simulink model "TorqueVect"  (R2022a)
settings: Solver=VariableStepAuto  StartTime=0.0  StopTime=32  RelTol=1e-3
PreLoadFcn:
  | run('Parameters\FSE_Parameters.m')
undefined symbols (not defined in the file): BRegenEnabledButton, canChannel, CyalphaLookUp, efficiency, Fz_curve, Fz_scaling_long, gearR, izz, jw, Kd, kd, Ki, ki, Kp, kp, l_f, l_r, lambda, m, Mz_max, N, N_lat, N_long, P_max, pid_kd_lat, pid_kd_long, pid_ki_lat, pid_ki_long, pid_kp_lat, pid_kp_long, R_max, rw, steerR, T_i_max, TC_Decr_Gas, TC_Derivative, TC_Incr_Gas, TC_On, TC_Relay_Off, TC_Relay_On, tireCornerStiffness, Ts, TV_On, TV_Override, velocity_lookup, velocity_lookup_lat, y_ref, yrr_scaling
libraries: simulink x218, slpidlib x135, CarMaker4SL x101, TractionControlLibrary x13, canmsglib x9, canlib x8, TorqueVectoringLibrary x6, simulink_extras x4, PedalConversionLibrary x3, PowerControlLibrary x1
(part 5 of 26)

== system TorqueVect/CarMaker/IPG Vehicle/PowerTrain/PTControl Example/PTControl_ALL_Speedgoat/New TC ==
  lim 1 : Inport
  lim 2 : Inport  Port=2
  lim 3 : Inport  Port=3
  lim 4 : Inport  Port=4
  vx : Inport  Port=5
  w_FL : Inport  Port=6
  w_FR : Inport  Port=7
  w_RL : Inport  Port=8
  w_RR : Inport  Port=9
  Front SR Target : Inport  Port=10
  Rear SR Target : Inport  Port=11
  P_TC : Inport  Port=12
  D_TC : Inport  Port=13
  enable_tc : Inport  Port=14
  rate_h : Inport  Port=15
  rate_l : Inport  Port=16
  Demux1 : Demux
  Gain : Gain  Gain=0.2032/13.39
  Rate Limiter Dynamic{,1..3} (4 alike) : simulink/Discontinuities/Rate Limiter Dynamic
  Reference Generator1 : Subsystem
  Saturation : Saturate  UpperLimit=inf  LowerLimit=0
  Subtract1 : Sum  Inputs=-+
  TC R1 : Subsystem
  TC R2 : Subsystem
  TC R3 : Subsystem
  TC R4 : Subsystem
  Vector Concatenate3 : Concatenate  NumInputs=4
  R1 Demand : Outport
  L1 Demand : Outport  Port=2
  R2 Demand : Outport  Port=3
  L2 Demand : Outport  Port=4
  wires:
  Reference Generator1/1(R1) -> TC R1/1(modified slip ratio reference)
  lim 1/1 -> TC R1/2(lim 1)
  Gain/1 -> Subtract1/2
  Vector Concatenate3/1 -> Gain/1  "omega"
  Subtract1/1 -> Demux1/1
  vx/1 -> Saturation/1
  TC R2/1(Control Effort 1) -> Rate Limiter Dynamic1/2  "MMotorL1Demand"
  w_RL/1 -> Vector Concatenate3/4
  w_RR/1 -> Vector Concatenate3/3
  w_FL/1 -> Vector Concatenate3/2
  w_FR/1 -> Vector Concatenate3/1
  Front SR Target/1 -> Reference Generator1/2(Front SR Target)
  Rear SR Target/1 -> Reference Generator1/3(Rear SR Target)
  lim 2/1 -> TC R2/2(lim 1)
  lim 3/1 -> TC R3/2(lim 1)
  lim 4/1 -> TC R4/2(lim 1)
  Reference Generator1/2(L1) -> TC R2/1(modified slip ratio reference)
  Reference Generator1/3(R2) -> TC R3/1(modified slip ratio reference)
  Reference Generator1/4(L2) -> TC R4/1(modified slip ratio reference)
  P_TC/1 -> TC R2/4(P_TC), TC R4/4(P_TC), TC R3/4(P_TC), TC R1/4(P_TC)
  D_TC/1 -> TC R2/5(D_TC), TC R4/5(D_TC), TC R3/5(D_TC), TC R1/5(D_TC)
  Demux1/1 -> TC R1/3(modified slip ratio measurement)
  Demux1/2 -> TC R2/3(modified slip ratio measurement)
  Demux1/3 -> TC R3/3(modified slip ratio measurement)
  Demux1/4 -> TC R4/3(modified slip ratio measurement)
  TC R1/1(Control Effort 1) -> Rate Limiter Dynamic/2  "MMotorR1Demand"
  Saturation/1 -> Subtract1/1, Reference Generator1/1(x2)
  TC R3/1(Control Effort 1) -> Rate Limiter Dynamic2/2
  TC R4/1(Control Effort 1) -> Rate Limiter Dynamic3/2
  enable_tc/1 -> TC R4/6(enable_tc), TC R2/6(enable_tc), TC R3/6(enable_tc), TC R1/6(enable_tc)
  Rate Limiter Dynamic/1 -> R1 Demand/1
  rate_h/1 -> Rate Limiter Dynamic3/1, Rate Limiter Dynamic2/1, Rate Limiter Dynamic1/1, Rate Limiter Dynamic/1
  rate_l/1 -> Rate Limiter Dynamic/3, Rate Limiter Dynamic3/3, Rate Limiter Dynamic2/3, Rate Limiter Dynamic1/3
  Rate Limiter Dynamic1/1 -> L1 Demand/1
  Rate Limiter Dynamic2/1 -> R2 Demand/1
  Rate Limiter Dynamic3/1 -> L2 Demand/1

== system TorqueVect/CarMaker/IPG Vehicle/PowerTrain/PTControl Example/PTControl_ALL_Speedgoat/PTC ==
  Constant2 : Constant
  Ground : Ground
  Mode_EngineDrive : Constant  Value=4
  Mux : Mux
  OperState_Driving : Constant  Value=4
  PTC MiscOut : Outport  VectorParamsAs1DForOutWhenUnconnected=off
  wires:
  Constant2/1 -> Mux/4  "Ignition"
  Mode_EngineDrive/1 -> Mux/3
  Ground/1 -> Mux/2  "OperationError"
  OperState_Driving/1 -> Mux/1
  Mux/1 -> PTC MiscOut/1

== system TorqueVect/CarMaker/IPG Vehicle/PowerTrain/PTControl Example/PTControl_ALL_Speedgoat/Subsystem ==
  VhclCtrl.PT : Inport
  PTControl_In : Inport  Port=2
  Bus Selector : BusSelector  OutputSignals=VhclCtrl Gas,VhclCtrl Brake
  Bus Selector1 : BusSelector  OutputSignals=Vel_B x,Vel_B y,Omega_B z,Acc_B x,Acc_B y
  Bus Selector2 : BusSelector  OutputSignals=PT:Motor.PT:Motor:Trq,PT:Motor.PT:Motor1:Trq,PT:Motor.PT:Motor2:Trq,PT:Motor.PT:Motor3:Trq,PT:Motor.PT:Motor:rotv,PT:Motor.PT:Motor1:rotv,PT:Motor.PT:Motor2:rotv,PT:Motor.PT:Motor3:rotv,Steer.Driver:Steer:Ang,Steer.Car:SteerAngle:FL,Steer.Car:SteerAngle:FR,PT:PwrSupply:HV1:Pwr
  CAN Configuration : canlib/CAN Configuration  BlockHandle=91645.0002  Device=MathWorks Virtual 1 (Channel 1)  DeviceMenu=MathWorks Virtual 1 (Channel 1)  ObjConstructor=canChannel('MathWorks', 'Virtual 1', 1)  BusSpeed=500000  EnableBitParameters=off  AckMode=Normal
      settings: SourceProductBaseCode=VN
  CAN Pack1 : canmsglib/CAN Pack  MsgList=(none)  MsgName=Wheel Torques  MsgIDType=Standard (11-bit identifier)  MsgIdentifier=600  MsgLength=8  Remote=off  ApplyMinMax=off  BusOutput=off  SignalInfo={ 'FL_Trq', '0', '16', 'LE', 'signed', 'Standard', '0', '1', '0', '-210', '210'; 'FR_Trq', '16', '16', 'LE', 'signed', 'Standard', '0', '1', '0', '-210', '210'; 'RL_Trq', '32', '16', 'LE', 'signed', 'Standard', '0', '1', '0', '-210', '210'; 'RR_Trq', '48', '16', 'LE', 'signed', 'Standard', '0', '1', '0', '-210', '210' }
      settings: SourceProductBaseCode=XP,ME,VN  DataFormat=manually specified signals
  CAN Pack2 : canmsglib/CAN Pack  MsgList=(none)  MsgName=Motor Speeds (rad/s)  MsgIDType=Standard (11-bit identifier)  MsgIdentifier=601  MsgLength=8  Remote=off  ApplyMinMax=off  BusOutput=off  SignalInfo={ 'FL_w', '0', '16', 'LE', 'signed', 'Standard', '0', '1', '0', '-32768', '32767'; 'FR_w', '16', '16', 'LE', 'signed', 'Standard', '0', '1', '0', '-32768', '32767'; 'RL_w', '32', '16', 'LE', 'signed', 'Standard', '0', '1', '0', '-32768', '32767'; 'RR_w', '48', '16', 'LE', 'signed', 'Standard', '0', '1', '0', '-32768', '32767' }
      settings: SourceProductBaseCode=XP,ME,VN  DataFormat=manually specified signals
  CAN Pack3 : canmsglib/CAN Pack  MsgList=(none)  MsgName=CAN Msg  MsgIDType=Standard (11-bit identifier)  MsgIdentifier=602  MsgLength=8  Remote=off  ApplyMinMax=off  BusOutput=off  SignalInfo={ 'Throttle', '0', '8', 'LE', 'unsigned', 'Standard', '0', '1', '0', '0', '100'; 'Brake', '8', '8', 'LE', 'unsigned', 'Standard', '0', '1', '0', '0', '100'; 'Steering Angle', '16', '16', 'LE', 'signed', 'Standard', '0', '1', '0', '-32768', '32767'; 'FL Angle', '32', '16', 'LE', 'signed', 'Standard', '0', '1', '0', '-32768', '32767'; 'FR Angle', '48', '16', 'LE', 'signed', 'Standard', '0', '1', '0', '-32768', '32767' }
      settings: SourceProductBaseCode=XP,ME,VN  DataFormat=manually specified signals
  CAN Pack4 : canmsglib/CAN Pack  MsgList=(none)  MsgName=CAN Msg  MsgIDType=Standard (11-bit identifier)  MsgIdentifier=603  MsgLength=8  Remote=off  ApplyMinMax=off  BusOutput=off  SignalInfo={ 'Vx', '0', '16', 'LE', 'signed', 'Standard', '0', '1', '0', '-32768', '32767'; 'Vy', '16', '16', 'LE', 'signed', 'Standard', '0', '1', '0', '-32768', '32767'; 'nYaw', '32', '16', 'LE', 'signed', 'Standard', '0', '1', '0', '-32768', '32767'; 'Power', '48', '16', 'LE', 'signed', 'Standard', '0', '1', '0', '-8000', '8000' }
      settings: SourceProductBaseCode=XP,ME,VN  DataFormat=manually specified signals
  CAN Pack5 : canmsglib/CAN Pack  Commented=on  MsgList=(none)  MsgName=CAN Msg  MsgIDType=Standard (11-bit identifier)  MsgIdentifier=605  MsgLength=8  Remote=off  ApplyMinMax=off  BusOutput=off  SignalInfo={ 'Pwr', '0', '32', 'LE', 'signed', 'Standard', '0', '1', '0', '-Inf', 'Inf' }
      settings: SourceProductBaseCode=XP,ME,VN  DataFormat=manually specified signals
  CAN Pack6 : canmsglib/CAN Pack  MsgList=(none)  MsgName=CAN Msg  MsgIDType=Standard (11-bit identifier)  MsgIdentifier=604  MsgLength=4  Remote=off  ApplyMinMax=off  BusOutput=off  SignalInfo={ 'Ax', '0', '16', 'LE', 'signed', 'Standard', '0', '1', '0', '-32768', '32767'; 'Ay', '16', '16', 'LE', 'signed', 'Standard', '0', '1', '0', '-32768', '32767' }
      settings: SourceProductBaseCode=XP,ME,VN  DataFormat=manually specified signals
  CAN Transmit1 : canlib/CAN Transmit  BlockHandle=92190.0002  Device=MathWorks Virtual 1 (Channel 1)  DeviceMenu=MathWorks Virtual 1 (Channel 1)  ObjConstructor=canChannel('MathWorks', 'Virtual 1', 1)  EnableEventTransmit=off  EnablePeriodicTransmit=on  MessagePeriod=0.01
      settings: SourceProductBaseCode=VN
  CAN Transmit2 : canlib/CAN Transmit  BlockHandle=92192.0002  Device=MathWorks Virtual 1 (Channel 1)  DeviceMenu=MathWorks Virtual 1 (Channel 1)  ObjConstructor=canChannel('MathWorks', 'Virtual 1', 1)  EnableEventTransmit=off  EnablePeriodicTransmit=on  MessagePeriod=0.01
      settings: SourceProductBaseCode=VN
  CAN Transmit3 : canlib/CAN Transmit  BlockHandle=92194.0002  Device=MathWorks Virtual 1 (Channel 1)  DeviceMenu=MathWorks Virtual 1 (Channel 1)  ObjConstructor=canChannel('MathWorks', 'Virtual 1', 1)  EnableEventTransmit=off  EnablePeriodicTransmit=on  MessagePeriod=0.01
      settings: SourceProductBaseCode=VN
  CAN Transmit4 : canlib/CAN Transmit  Commented=on  BlockHandle=92196.0011  Device=MathWorks Virtual 1 (Channel 1)  DeviceMenu=MathWorks Virtual 1 (Channel 1)  ObjConstructor=canChannel('MathWorks', 'Virtual 1', 1)  EnableEventTransmit=off  EnablePeriodicTransmit=on  MessagePeriod=0.01
      settings: SourceProductBaseCode=VN
  CAN Transmit5 : canlib/CAN Transmit  BlockHandle=92198.0002  Device=MathWorks Virtual 1 (Channel 1)  DeviceMenu=MathWorks Virtual 1 (Channel 1)  ObjConstructor=canChannel('MathWorks', 'Virtual 1', 1)  EnableEventTransmit=off  EnablePeriodicTransmit=on  MessagePeriod=0.01
      settings: SourceProductBaseCode=VN
  CAN Transmit6 : canlib/CAN Transmit  BlockHandle=92200.0002  Device=MathWorks Virtual 1 (Channel 1)  DeviceMenu=MathWorks Virtual 1 (Channel 1)  ObjConstructor=canChannel('MathWorks', 'Virtual 1', 1)  EnableEventTransmit=off  EnablePeriodicTransmit=on  MessagePeriod=0.01
      settings: SourceProductBaseCode=VN
  Gain{,1..3} (4 alike) : Gain  Gain=10
  Gain10 : Gain  Gain=1000
  Gain11 : Gain  Gain=1000
  Gain12 : Gain  Gain=1000
  Gain{8..9,13..15,17..18} (7 alike) : Gain  Gain=100
  Gain16 : Gain  Gain=1/10
  Gain{4..7} (4 alike) : Gain  Gain=30/pi
  Inertial Sensor : CarMaker4SL/Sensors/Inertial Sensor  xname=Param_B00  xstime=Continuous
      settings: SourceProductName=CarMaker4SL
  Rate Transition{,1..18} (19 alike) : RateTransition  OutPortSampleTime=0.001
  Subsystem : Subsystem
  Terminator : Terminator
  <PT:Motor:Trq> : Outport
  <PT:Motor1:Trq> : Outport  Port=2
  <PT:Motor2:Trq> : Outport  Port=3
  <PT:Motor3:Trq> : Outport  Port=4
  wires:
  Inertial Sensor/1 -> Terminator/1
  Inertial Sensor/2 -> Bus Selector1/1
  PTControl_In/1 -> Bus Selector2/1
  VhclCtrl.PT/1 -> Bus Selector/1
  Bus Selector2/1 -> Rate Transition/1  "<PT:Motor:Trq>"
  Bus Selector2/2 -> Rate Transition1/1  "<PT:Motor1:Trq>"
  Bus Selector2/3 -> Rate Transition2/1  "<PT:Motor2:Trq>"
  Bus Selector2/4 -> Rate Transition3/1  "<PT:Motor3:Trq>"
  Bus Selector2/5 -> Rate Transition4/1  "<PT:Motor:rotv>"
  Bus Selector2/6 -> Rate Transition5/1  "<PT:Motor1:rotv>"
  Bus Selector2/7 -> Rate Transition6/1  "<PT:Motor2:rotv>"
  Bus Selector2/8 -> Rate Transition7/1  "<PT:Motor3:rotv>"
  Bus Selector/2 -> Rate Transition9/1  "<VhclCtrl Brake>"
  Bus Selector2/9 -> Rate Transition10/1  "<Driver:Steer:Ang>"
  Bus Selector2/10 -> Rate Transition11/1  "<Car:SteerAngle:FL>"
  Bus Selector2/11 -> Rate Transition12/1  "<Car:SteerAngle:FR>"
  Bus Selector1/1 -> Rate Transition14/1  "<Vel_B x>"
  Bus Selector1/2 -> Rate Transition15/1  "<Vel_B y>"
  Bus Selector1/3 -> Rate Transition16/1  "<Omega_B z>"
  Bus Selector2/12 -> Rate Transition13/1  "<PT:PwrSupply:HV1:Pwr>"
  CAN Pack1/1 -> CAN Transmit1/1
  CAN Pack2/1 -> CAN Transmit2/1
  CAN Pack3/1 -> CAN Transmit3/1
  CAN Pack5/1 -> CAN Transmit4/1
  CAN Pack4/1 -> CAN Transmit5/1
  Subsystem/1(Out1) -> <PT:Motor:Trq>/1
  Subsystem/2(Out2) -> <PT:Motor1:Trq>/1
  Subsystem/3(Out3) -> <PT:Motor2:Trq>/1
  Subsystem/4(Out4) -> <PT:Motor3:Trq>/1
  Rate Transition/1 -> Gain/1
  Rate Transition1/1 -> Gain1/1
  Rate Transition2/1 -> Gain2/1
  Rate Transition3/1 -> Gain3/1
  Rate Transition4/1 -> Gain4/1
  Rate Transition5/1 -> Gain5/1
  Rate Transition6/1 -> Gain6/1
  Rate Transition7/1 -> Gain7/1
  Rate Transition9/1 -> Gain9/1
  Rate Transition10/1 -> Gain10/1
  Rate Transition11/1 -> Gain11/1
  Rate Transition12/1 -> Gain12/1
  Rate Transition13/1 -> Gain16/1
  Rate Transition14/1 -> Gain13/1
  Rate Transition15/1 -> Gain14/1
  Rate Transition16/1 -> Gain15/1
  Bus Selector/1 -> Rate Transition8/1  "<VhclCtrl Gas>"
  Rate Transition8/1 -> Gain8/1
  Gain/1 -> CAN Pack1/1
  Gain1/1 -> CAN Pack1/2
  Gain2/1 -> CAN Pack1/3
  Gain3/1 -> CAN Pack1/4
  Gain6/1 -> CAN Pack2/3
  Gain5/1 -> CAN Pack2/2
  Gain7/1 -> CAN Pack2/4
  Gain4/1 -> CAN Pack2/1
  Gain8/1 -> CAN Pack3/1
  Gain9/1 -> CAN Pack3/2
  Gain10/1 -> CAN Pack3/3
  Gain11/1 -> CAN Pack3/4
  Gain12/1 -> CAN Pack3/5
  Gain13/1 -> CAN Pack4/1
  Gain14/1 -> CAN Pack4/2
  Gain15/1 -> CAN Pack4/3
  Gain16/1 -> CAN Pack4/4, CAN Pack5/1
  Bus Selector1/5 -> Rate Transition18/1  "<Acc_B y>"
  Rate Transition18/1 -> Gain17/1
  Rate Transition17/1 -> Gain18/1
  Gain17/1 -> CAN Pack6/2
  Gain18/1 -> CAN Pack6/1
  Bus Selector1/4 -> Rate Transition17/1  "<Acc_B x>"
  CAN Pack6/1 -> CAN Transmit6/1

== system TorqueVect/CarMaker/IPG Vehicle/PowerTrain/PTControl Example/PTControl_In1/CreateBus PTC Battery ==
  In : Inport
  BusCreator : BusCreator  Inputs=14
  Demux : Demux  Outputs=14
      settings: DisplayOption=none
  Out : Outport  VectorParamsAs1DForOutWhenUnconnected=off
  wires:
  In/1 -> Demux/1
  BusCreator/1 -> Out/1
  Demux/1 -> BusCreator/1  "PTC BattLVIn SOC"
  Demux/2 -> BusCreator/2  "PTC BattLVIn SOH"
  Demux/3 -> BusCreator/3  "PTC BattLVIn Current"
  Demux/4 -> BusCreator/4  "PTC BattLVIn AOC"
  Demux/5 -> BusCreator/5  "PTC BattLVIn Temp"
  Demux/6 -> BusCreator/6  "PTC BattLVIn Energy"
  Demux/7 -> BusCreator/7  "PTC BattLVIn Pwr_max"
  Demux/8 -> BusCreator/8  "PTC BattHVIn SOC"
  Demux/9 -> BusCreator/9  "PTC BattHVIn SOH"
  Demux/10 -> BusCreator/10  "PTC BattHVIn Current"
  Demux/11 -> BusCreator/11  "PTC BattHVIn AOC"
  Demux/12 -> BusCreator/12  "PTC BattHVIn Temp"
  Demux/13 -> BusCreator/13  "PTC BattHVIn Energy"
  Demux/14 -> BusCreator/14  "PTC BattHVIn Pwr_max"

== system TorqueVect/CarMaker/IPG Vehicle/PowerTrain/PTControl Example/PTControl_In1/CreateBus PTC ClutchIn ==
  In : Inport
  BusCreator : BusCreator  Inputs=6
  Demux : Demux  Outputs=6
      settings: DisplayOption=none
  Out : Outport  VectorParamsAs1DForOutWhenUnconnected=off
  wires:
  In/1 -> Demux/1
  BusCreator/1 -> Out/1
  Demux/1 -> BusCreator/1  "PTC ClutchIn Pos"
  Demux/2 -> BusCreator/2  "PTC ClutchIn rotv_in"
  Demux/3 -> BusCreator/3  "PTC ClutchIn rotv_out"
  Demux/4 -> BusCreator/4  "PTC ClutchIn Trq_in"
  Demux/5 -> BusCreator/5  "PTC ClutchIn Trq_out"
  Demux/6 -> BusCreator/6  "PTC ClutchIn i_TrqIn2Out"

== system TorqueVect/CarMaker/IPG Vehicle/PowerTrain/PTControl Example/PTControl_In1/CreateBus PTC Control Units ==
  In : Inport
  BusCreator : BusCreator  Inputs=4
  Demux : Demux
      settings: DisplayOption=none
  Out : Outport  VectorParamsAs1DForOutWhenUnconnected=off
  wires:
  In/1 -> Demux/1
  BusCreator/1 -> Out/1
  Demux/1 -> BusCreator/1  "PTC ECU_Status"
  Demux/2 -> BusCreator/2  "PTC MCU_Status"
  Demux/3 -> BusCreator/3  "PTC TCU_Status"
  Demux/4 -> BusCreator/4  "PTC BCU_Status"

== system TorqueVect/CarMaker/IPG Vehicle/PowerTrain/PTControl Example/PTControl_In1/CreateBus PTC DriveSrcIn ==
  In : Inport
  BusCreator : BusCreator  Inputs=4
  Demux : Demux
      settings: DisplayOption=none
  Out : Outport  VectorParamsAs1DForOutWhenUnconnected=off
  wires:
  In/1 -> Demux/1
  BusCreator/1 -> Out/1
  Demux/1 -> BusCreator/1  "PTC DriveSrcIn_d0 Trq_DriveSrc_trg"
  Demux/2 -> BusCreator/2  "PTC DriveSrcIn_d1 Trq_DriveSrc_trg"
  Demux/3 -> BusCreator/3  "PTC DriveSrcIn_d2 Trq_DriveSrc_trg"
  Demux/4 -> BusCreator/4  "PTC DriveSrcIn_d3 Trq_DriveSrc_trg"

== system TorqueVect/CarMaker/IPG Vehicle/PowerTrain/PTControl Example/PTControl_In1/CreateBus PTC EngineIn ==
  In : Inport
  BusCreator : BusCreator  Inputs=7
  Demux : Demux  Outputs=7
      settings: DisplayOption=none
  Out : Outport  VectorParamsAs1DForOutWhenUnconnected=off
  wires:
  In/1 -> Demux/1
  BusCreator/1 -> Out/1
  Demux/1 -> BusCreator/1  "PTC EngineIn Engine_on"
  Demux/2 -> BusCreator/2  "PTC EngineIn rotv"
  Demux/3 -> BusCreator/3  "PTC EngineIn Trq"
  Demux/4 -> BusCreator/4  "PTC EngineIn TrqDrag"
  Demux/5 -> BusCreator/5  "PTC EngineIn TrqFull"
  Demux/6 -> BusCreator/6  "PTC EngineIn TrqOpt"
  Demux/7 -> BusCreator/7  "PTC EngineIn FuelFlow"

== system TorqueVect/CarMaker/IPG Vehicle/PowerTrain/PTControl Example/PTControl_In1/CreateBus PTC GearBoxIn ==
  In : Inport
  BusCreator : BusCreator  Inputs=20
  Demux : Demux  Outputs=20
      settings: DisplayOption=none
  Out : Outport  VectorParamsAs1DForOutWhenUnconnected=off
  wires:
  In/1 -> Demux/1
  BusCreator/1 -> Out/1
  Demux/1 -> BusCreator/1  "PTC GearBoxIn GearNo"
  Demux/2 -> BusCreator/2  "PTC GearBoxIn GearNo_dis"
  Demux/3 -> BusCreator/3  "PTC GearBoxIn Trq_DriveSrc_trg"
  Demux/4 -> BusCreator/4  "PTC GearBoxIn i"
  Demux/5 -> BusCreator/5  "PTC GearBoxIn rotv_in"
  Demux/6 -> BusCreator/6  "PTC GearBoxIn rotv_out"
  Demux/7 -> BusCreator/7  "PTC GearBoxIn Trq_in"
  Demux/8 -> BusCreator/8  "PTC GearBoxIn Trq_out"
  Demux/9 -> BusCreator/9  "PTC GearBoxIn Clutch Pos"
  Demux/10 -> BusCreator/10  "PTC GearBoxIn Clutch rotv_in"
  Demux/11 -> BusCreator/11  "PTC GearBoxIn Clutch rotv_out"
  Demux/12 -> BusCreator/12  "PTC GearBoxIn Clutch Trq_in"
  Demux/13 -> BusCreator/13  "PTC GearBoxIn Clutch Trq_out"
  Demux/14 -> BusCreator/14  "PTC GearBoxIn Clutch i_TrqIn2Out"
  Demux/15 -> BusCreator/15  "PTC GearBoxIn Clutch_dis Pos"
  Demux/16 -> BusCreator/16  "PTC GearBoxIn Clutch_dis rotv_in"
  Demux/17 -> BusCreator/17  "PTC GearBoxIn Clutch_dis rotv_out"
  Demux/18 -> BusCreator/18  "PTC GearBoxIn Clutch_dis Trq_in"
  Demux/19 -> BusCreator/19  "PTC GearBoxIn Clutch_dis Trq_out"
  Demux/20 -> BusCreator/20  "PTC GearBoxIn Clutch_dis i_TrqIn2Out"

== system TorqueVect/CarMaker/IPG Vehicle/PowerTrain/PTControl Example/PTControl_In1/CreateBus PTC GearBoxM_In0 ==
  In : Inport
  BusCreator : BusCreator  Inputs=20
  Demux : Demux  Outputs=20
      settings: DisplayOption=none
  Out : Outport  VectorParamsAs1DForOutWhenUnconnected=off
  wires:
  In/1 -> Demux/1
  BusCreator/1 -> Out/1
  Demux/1 -> BusCreator/1  "PTC GearBoxM_In0 GearNo"
  Demux/2 -> BusCreator/2  "PTC GearBoxM_In0 GearNo_dis"
  Demux/3 -> BusCreator/3  "PTC GearBoxM_In0 Trq_DriveSrc_trg"
  Demux/4 -> BusCreator/4  "PTC GearBoxM_In0 i"
  Demux/5 -> BusCreator/5  "PTC GearBoxM_In0 rotv_in"
  Demux/6 -> BusCreator/6  "PTC GearBoxM_In0 rotv_out"
  Demux/7 -> BusCreator/7  "PTC GearBoxM_In0 Trq_in"
  Demux/8 -> BusCreator/8  "PTC GearBoxM_In0 Trq_out"
  Demux/9 -> BusCreator/9  "PTC GearBoxM_In0 Clutch Pos"
  Demux/10 -> BusCreator/10  "PTC GearBoxM_In0 Clutch rotv_in"
  Demux/11 -> BusCreator/11  "PTC GearBoxM_In0 Clutch rotv_out"
  Demux/12 -> BusCreator/12  "PTC GearBoxM_In0 Clutch Trq_in"
  Demux/13 -> BusCreator/13  "PTC GearBoxM_In0 Clutch Trq_out"
  Demux/14 -> BusCreator/14  "PTC GearBoxM_In0 Clutch i_TrqIn2Out"
  Demux/15 -> BusCreator/15  "PTC GearBoxM_In0 Clutch_dis Pos"
  Demux/16 -> BusCreator/16  "PTC GearBoxM_In0 Clutch_dis rotv_in"
  Demux/17 -> BusCreator/17  "PTC GearBoxM_In0 Clutch_dis rotv_out"
  Demux/18 -> BusCreator/18  "PTC GearBoxM_In0 Clutch_dis Trq_in"
  Demux/19 -> BusCreator/19  "PTC GearBoxM_In0 Clutch_dis Trq_out"
  Demux/20 -> BusCreator/20  "PTC GearBoxM_In0 Clutch_dis i_TrqIn2Out"

== system TorqueVect/CarMaker/IPG Vehicle/PowerTrain/PTControl Example/PTControl_In1/CreateBus PTC GearBoxM_In1 ==
  In : Inport
  BusCreator : BusCreator  Inputs=20
  Demux : Demux  Outputs=20
      settings: DisplayOption=none
  Out : Outport  VectorParamsAs1DForOutWhenUnconnected=off
  wires:
  In/1 -> Demux/1
  BusCreator/1 -> Out/1
  Demux/1 -> BusCreator/1  "PTC GearBoxM_In1 GearNo"
  Demux/2 -> BusCreator/2  "PTC GearBoxM_In1 GearNo_dis"
  Demux/3 -> BusCreator/3  "PTC GearBoxM_In1 Trq_DriveSrc_trg"
  Demux/4 -> BusCreator/4  "PTC GearBoxM_In1 i"
  Demux/5 -> BusCreator/5  "PTC GearBoxM_In1 rotv_in"
  Demux/6 -> BusCreator/6  "PTC GearBoxM_In1 rotv_out"
  Demux/7 -> BusCreator/7  "PTC GearBoxM_In1 Trq_in"
  Demux/8 -> BusCreator/8  "PTC GearBoxM_In1 Trq_out"
  Demux/9 -> BusCreator/9  "PTC GearBoxM_In1 Clutch Pos"
  Demux/10 -> BusCreator/10  "PTC GearBoxM_In1 Clutch rotv_in"
  Demux/11 -> BusCreator/11  "PTC GearBoxM_In1 Clutch rotv_out"
  Demux/12 -> BusCreator/12  "PTC GearBoxM_In1 Clutch Trq_in"
  Demux/13 -> BusCreator/13  "PTC GearBoxM_In1 Clutch Trq_out"
  Demux/14 -> BusCreator/14  "PTC GearBoxM_In1 Clutch i_TrqIn2Out"
  Demux/15 -> BusCreator/15  "PTC GearBoxM_In1 Clutch_dis Pos"
  Demux/16 -> BusCreator/16  "PTC GearBoxM_In1 Clutch_dis rotv_in"
  Demux/17 -> BusCreator/17  "PTC GearBoxM_In1 Clutch_dis rotv_out"
  Demux/18 -> BusCreator/18  "PTC GearBoxM_In1 Clutch_dis Trq_in"
  Demux/19 -> BusCreator/19  "PTC GearBoxM_In1 Clutch_dis Trq_out"
  Demux/20 -> BusCreator/20  "PTC GearBoxM_In1 Clutch_dis i_TrqIn2Out"

== system TorqueVect/CarMaker/IPG Vehicle/PowerTrain/PTControl Example/PTControl_In1/CreateBus PTC GearBoxM_In2 ==
  In : Inport
  BusCreator : BusCreator  Inputs=20
  Demux : Demux  Outputs=20
      settings: DisplayOption=none
  Out : Outport  VectorParamsAs1DForOutWhenUnconnected=off
  wires:
  In/1 -> Demux/1
  BusCreator/1 -> Out/1
  Demux/1 -> BusCreator/1  "PTC GearBoxM_In2 GearNo"
  Demux/2 -> BusCreator/2  "PTC GearBoxM_In2 GearNo_dis"
  Demux/3 -> BusCreator/3  "PTC GearBoxM_In2 Trq_DriveSrc_trg"
  Demux/4 -> BusCreator/4  "PTC GearBoxM_In2 i"
  Demux/5 -> BusCreator/5  "PTC GearBoxM_In2 rotv_in"
  Demux/6 -> BusCreator/6  "PTC GearBoxM_In2 rotv_out"
  Demux/7 -> BusCreator/7  "PTC GearBoxM_In2 Trq_in"
  Demux/8 -> BusCreator/8  "PTC GearBoxM_In2 Trq_out"
  Demux/9 -> BusCreator/9  "PTC GearBoxM_In2 Clutch Pos"
  Demux/10 -> BusCreator/10  "PTC GearBoxM_In2 Clutch rotv_in"
  Demux/11 -> BusCreator/11  "PTC GearBoxM_In2 Clutch rotv_out"
  Demux/12 -> BusCreator/12  "PTC GearBoxM_In2 Clutch Trq_in"
  Demux/13 -> BusCreator/13  "PTC GearBoxM_In2 Clutch Trq_out"
  Demux/14 -> BusCreator/14  "PTC GearBoxM_In2 Clutch i_TrqIn2Out"
  Demux/15 -> BusCreator/15  "PTC GearBoxM_In2 Clutch_dis Pos"
  Demux/16 -> BusCreator/16  "PTC GearBoxM_In2 Clutch_dis rotv_in"
  Demux/17 -> BusCreator/17  "PTC GearBoxM_In2 Clutch_dis rotv_out"
  Demux/18 -> BusCreator/18  "PTC GearBoxM_In2 Clutch_dis Trq_in"
  Demux/19 -> BusCreator/19  "PTC GearBoxM_In2 Clutch_dis Trq_out"
  Demux/20 -> BusCreator/20  "PTC GearBoxM_In2 Clutch_dis i_TrqIn2Out"

== system TorqueVect/CarMaker/IPG Vehicle/PowerTrain/PTControl Example/PTControl_In1/CreateBus PTC GearBoxM_In3 ==
  In : Inport
  BusCreator : BusCreator  Inputs=20
  Demux : Demux  Outputs=20
      settings: DisplayOption=none
  Out : Outport  VectorParamsAs1DForOutWhenUnconnected=off
  wires:
  In/1 -> Demux/1
  BusCreator/1 -> Out/1
  Demux/1 -> BusCreator/1  "PTC GearBoxM_In3 GearNo"
  Demux/2 -> BusCreator/2  "PTC GearBoxM_In3 GearNo_dis"
  Demux/3 -> BusCreator/3  "PTC GearBoxM_In3 Trq_DriveSrc_trg"
  Demux/4 -> BusCreator/4  "PTC GearBoxM_In3 i"
  Demux/5 -> BusCreator/5  "PTC GearBoxM_In3 rotv_in"
  Demux/6 -> BusCreator/6  "PTC GearBoxM_In3 rotv_out"
  Demux/7 -> BusCreator/7  "PTC GearBoxM_In3 Trq_in"
  Demux/8 -> BusCreator/8  "PTC GearBoxM_In3 Trq_out"
  Demux/9 -> BusCreator/9  "PTC GearBoxM_In3 Clutch Pos"
  Demux/10 -> BusCreator/10  "PTC GearBoxM_In3 Clutch rotv_in"
  Demux/11 -> BusCreator/11  "PTC GearBoxM_In3 Clutch rotv_out"
  Demux/12 -> BusCreator/12  "PTC GearBoxM_In3 Clutch Trq_in"
  Demux/13 -> BusCreator/13  "PTC GearBoxM_In3 Clutch Trq_out"
  Demux/14 -> BusCreator/14  "PTC GearBoxM_In3 Clutch i_TrqIn2Out"
  Demux/15 -> BusCreator/15  "PTC GearBoxM_In3 Clutch_dis Pos"
  Demux/16 -> BusCreator/16  "PTC GearBoxM_In3 Clutch_dis rotv_in"
  Demux/17 -> BusCreator/17  "PTC GearBoxM_In3 Clutch_dis rotv_out"
  Demux/18 -> BusCreator/18  "PTC GearBoxM_In3 Clutch_dis Trq_in"
  Demux/19 -> BusCreator/19  "PTC GearBoxM_In3 Clutch_dis Trq_out"
  Demux/20 -> BusCreator/20  "PTC GearBoxM_In3 Clutch_dis i_TrqIn2Out"

== system TorqueVect/CarMaker/IPG Vehicle/PowerTrain/PTControl Example/PTControl_In1/CreateBus PTC ISGIn ==
  In : Inport
  BusCreator : BusCreator  Inputs=9
  Demux : Demux  Outputs=9
      settings: DisplayOption=none
  Out : Outport  VectorParamsAs1DForOutWhenUnconnected=off
  wires:
  In/1 -> Demux/1
  BusCreator/1 -> Out/1
  Demux/1 -> BusCreator/1  "PTC ISGIn rotv"
  Demux/2 -> BusCreator/2  "PTC ISGIn Trq"
  Demux/3 -> BusCreator/3  "PTC ISGIn TrqMot_max"
  Demux/4 -> BusCreator/4  "PTC ISGIn TrqGen_max"
  Demux/5 -> BusCreator/5  "PTC ISGIn PwrElec"
  Demux/6 -> BusCreator/6  "PTC ISGIn i_M2W_FL"
  Demux/7 -> BusCreator/7  "PTC ISGIn i_M2W_FR"
  Demux/8 -> BusCreator/8  "PTC ISGIn i_M2W_RL"
  Demux/9 -> BusCreator/9  "PTC ISGIn i_M2W_RR"

== system TorqueVect/CarMaker/IPG Vehicle/PowerTrain/PTControl Example/PTControl_In1/CreateBus PTC MotorIn0 ==
  In : Inport
  BusCreator : BusCreator  Inputs=9
  Demux : Demux  Outputs=9
      settings: DisplayOption=none
  Out : Outport  VectorParamsAs1DForOutWhenUnconnected=off
  wires:
  In/1 -> Demux/1
  BusCreator/1 -> Out/1
  Demux/1 -> BusCreator/1  "PTC MotorIn0 rotv"
  Demux/2 -> BusCreator/2  "PTC MotorIn0 Trq"
  Demux/3 -> BusCreator/3  "PTC MotorIn0 TrqMot_max"
  Demux/4 -> BusCreator/4  "PTC MotorIn0 TrqGen_max"
  Demux/5 -> BusCreator/5  "PTC MotorIn0 PwrElec"
  Demux/6 -> BusCreator/6  "PTC MotorIn0 i_M2W_FL"
  Demux/7 -> BusCreator/7  "PTC MotorIn0 i_M2W_FR"
  Demux/8 -> BusCreator/8  "PTC MotorIn0 i_M2W_RL"
  Demux/9 -> BusCreator/9  "PTC MotorIn0 i_M2W_RR"

== system TorqueVect/CarMaker/IPG Vehicle/PowerTrain/PTControl Example/PTControl_In1/CreateBus PTC MotorIn1 ==
  In : Inport
  BusCreator : BusCreator  Inputs=9
  Demux : Demux  Outputs=9
      settings: DisplayOption=none
  Out : Outport  VectorParamsAs1DForOutWhenUnconnected=off
  wires:
  In/1 -> Demux/1
  BusCreator/1 -> Out/1
  Demux/1 -> BusCreator/1  "PTC MotorIn1 rotv"
  Demux/2 -> BusCreator/2  "PTC MotorIn1 Trq"
  Demux/3 -> BusCreator/3  "PTC MotorIn1 TrqMot_max"
  Demux/4 -> BusCreator/4  "PTC MotorIn1 TrqGen_max"
  Demux/5 -> BusCreator/5  "PTC MotorIn1 PwrElec"
  Demux/6 -> BusCreator/6  "PTC MotorIn1 i_M2W_FL"
  Demux/7 -> BusCreator/7  "PTC MotorIn1 i_M2W_FR"
  Demux/8 -> BusCreator/8  "PTC MotorIn1 i_M2W_RL"
  Demux/9 -> BusCreator/9  "PTC MotorIn1 i_M2W_RR"

== system TorqueVect/CarMaker/IPG Vehicle/PowerTrain/PTControl Example/PTControl_In1/CreateBus PTC MotorIn2 ==
  In : Inport
  BusCreator : BusCreator  Inputs=9
  Demux : Demux  Outputs=9
      settings: DisplayOption=none
  Out : Outport  VectorParamsAs1DForOutWhenUnconnected=off
  wires:
  In/1 -> Demux/1
  BusCreator/1 -> Out/1
  Demux/1 -> BusCreator/1  "PTC MotorIn2 rotv"
  Demux/2 -> BusCreator/2  "PTC MotorIn2 Trq"
  Demux/3 -> BusCreator/3  "PTC MotorIn2 TrqMot_max"
  Demux/4 -> BusCreator/4  "PTC MotorIn2 TrqGen_max"
  Demux/5 -> BusCreator/5  "PTC MotorIn2 PwrElec"
  Demux/6 -> BusCreator/6  "PTC MotorIn2 i_M2W_FL"
  Demux/7 -> BusCreator/7  "PTC MotorIn2 i_M2W_FR"
  Demux/8 -> BusCreator/8  "PTC MotorIn2 i_M2W_RL"
  Demux/9 -> BusCreator/9  "PTC MotorIn2 i_M2W_RR"

== system TorqueVect/CarMaker/IPG Vehicle/PowerTrain/PTControl Example/PTControl_In1/CreateBus PTC MotorIn3 ==
  In : Inport
  BusCreator : BusCreator  Inputs=9
  Demux : Demux  Outputs=9
      settings: DisplayOption=none
  Out : Outport  VectorParamsAs1DForOutWhenUnconnected=off
  wires:
  In/1 -> Demux/1
  BusCreator/1 -> Out/1
  Demux/1 -> BusCreator/1  "PTC MotorIn3 rotv"
  Demux/2 -> BusCreator/2  "PTC MotorIn3 Trq"
  Demux/3 -> BusCreator/3  "PTC MotorIn3 TrqMot_max"
  Demux/4 -> BusCreator/4  "PTC MotorIn3 TrqGen_max"
  Demux/5 -> BusCreator/5  "PTC MotorIn3 PwrElec"
  Demux/6 -> BusCreator/6  "PTC MotorIn3 i_M2W_FL"
  Demux/7 -> BusCreator/7  "PTC MotorIn3 i_M2W_FR"
  Demux/8 -> BusCreator/8  "PTC MotorIn3 i_M2W_RL"
  Demux/9 -> BusCreator/9  "PTC MotorIn3 i_M2W_RR"

== system TorqueVect/CarMaker/IPG Vehicle/PowerTrain/PTControl Example/PTControl_In1/CreateBus PTC PwrSupplyIn ==
  In : Inport
  BusCreator : BusCreator  Inputs=12
  Demux : Demux  Outputs=12
      settings: DisplayOption=none
  Out : Outport  VectorParamsAs1DForOutWhenUnconnected=off
  wires:
  In/1 -> Demux/1
  BusCreator/1 -> Out/1
  Demux/1 -> BusCreator/1  "PTC PwrSupplyIn Pwr_LV"
  Demux/2 -> BusCreator/2  "PTC PwrSupplyIn Pwr_HV1"
  Demux/3 -> BusCreator/3  "PTC PwrSupplyIn Pwr_HV2"
  Demux/4 -> BusCreator/4  "PTC PwrSupplyIn Voltage_LV"
  Demux/5 -> BusCreator/5  "PTC PwrSupplyIn Voltage_HV1"
  Demux/6 -> BusCreator/6  "PTC PwrSupplyIn Voltage_HV2"
  Demux/7 -> BusCreator/7  "PTC PwrSupplyIn Pwr_HV1toLV"
  Demux/8 -> BusCreator/8  "PTC PwrSupplyIn Pwr_HV1toHV2"
  Demux/9 -> BusCreator/9  "PTC PwrSupplyIn Pwr_HV1toLV_max"
  Demux/10 -> BusCreator/10  "PTC PwrSupplyIn Pwr_HV1toHV2_max"
  Demux/11 -> BusCreator/11  "PTC PwrSupplyIn Eta_HV1toLV"
  Demux/12 -> BusCreator/12  "PTC PwrSupplyIn Eta_HV1toHV2"

== system TorqueVect/CarMaker/IPG Vehicle/PowerTrain/PTControl Example/PTControl_In1/CreateBus PTC Vehicle Ctrl ==
  In : Inport
  BusCreator : BusCreator  Inputs=8
  Demux : Demux  Outputs=8
      settings: DisplayOption=none
  Out : Outport  VectorParamsAs1DForOutWhenUnconnected=off
  wires:
  In/1 -> Demux/1
  BusCreator/1 -> Out/1
  Demux/1 -> BusCreator/1  "PTC Key"
  Demux/2 -> BusCreator/2  "PTC SST"
  Demux/3 -> BusCreator/3  "PTC SelectorCtrl"
  Demux/4 -> BusCreator/4  "PTC GearNoTrg"
  Demux/5 -> BusCreator/5  "PTC Clutch"
  Demux/6 -> BusCreator/6  "PTC Gas"
  Demux/7 -> BusCreator/7  "PTC Brake"
  Demux/8 -> BusCreator/8  "PTC Velocity"

== system TorqueVect/CarMaker/IPG Vehicle/PowerTrain/PTControl Example/PTControl_In1/CreateBus PTC WheelIn ==
  In : Inport
  BusCreator : BusCreator  Inputs=4
  Demux : Demux
      settings: DisplayOption=none
  Out : Outport  VectorParamsAs1DForOutWhenUnconnected=off
  wires:
  In/1 -> Demux/1
  BusCreator/1 -> Out/1
  Demux/1 -> BusCreator/1  "PTC WheelIn_FL Trq_BrakeReg_trg"
  Demux/2 -> BusCreator/2  "PTC WheelIn_FR Trq_BrakeReg_trg"
  Demux/3 -> BusCreator/3  "PTC WheelIn_RL Trq_BrakeReg_trg"
  Demux/4 -> BusCreator/4  "PTC WheelIn_RR Trq_BrakeReg_trg"

== system TorqueVect/CarMaker/IPG Vehicle/PowerTrain/PTControl Example/PTControl_In1/CreateBus PTC_Cfg Battery ==
  In : Inport
  BusCreator : BusCreator  Inputs=8
  Demux : Demux  Outputs=8
      settings: DisplayOption=none
  Out : Outport  VectorParamsAs1DForOutWhenUnconnected=off
  wires:
  In/1 -> Demux/1
  BusCreator/1 -> Out/1
  Demux/1 -> BusCreator/1  "PTC_Cfg BattLV SOC_min"
  Demux/2 -> BusCreator/2  "PTC_Cfg BattLV SOC_max"
  Demux/3 -> BusCreator/3  "PTC_Cfg BattLV Capacity"
  Demux/4 -> BusCreator/4  "PTC_Cfg BattLV Voltage"
  Demux/5 -> BusCreator/5  "PTC_Cfg BattHV SOC_min"
  Demux/6 -> BusCreator/6  "PTC_Cfg BattHV SOC_max"
  Demux/7 -> BusCreator/7  "PTC_Cfg BattHV Capacity"
  Demux/8 -> BusCreator/8  "PTC_Cfg BattHV Voltage"

== system TorqueVect/CarMaker/IPG Vehicle/PowerTrain/PTControl Example/PTControl_In1/CreateBus PTC_Cfg Engine ==
  In : Inport
  BusCreator : BusCreator  Inputs=4
  Demux : Demux
      settings: DisplayOption=none
  Out : Outport  VectorParamsAs1DForOutWhenUnconnected=off
  wires:
  In/1 -> Demux/1
  BusCreator/1 -> Out/1
  Demux/1 -> BusCreator/1  "PTC_Cfg Engine Fuel_l2kWh"
  Demux/2 -> BusCreator/2  "PTC_Cfg Engine rotv_max"
  Demux/3 -> BusCreator/3  "PTC_Cfg Engine rotv_idle"
  Demux/4 -> BusCreator/4  "PTC_Cfg Engine rotv_opt"

== system TorqueVect/CarMaker/IPG Vehicle/PowerTrain/PTControl Example/PTControl_In1/CreateBus PTC_Cfg GearBox ==
  In : Inport
  BusCreator : BusCreator  Inputs=38
  Demux : Demux  Outputs=38
      settings: DisplayOption=none
  Out : Outport  VectorParamsAs1DForOutWhenUnconnected=off
  wires:
  In/1 -> Demux/1
  BusCreator/1 -> Out/1
  Demux/1 -> BusCreator/1  "PTC_Cfg GearBox GBKind"
  Demux/2 -> BusCreator/2  "PTC_Cfg GearBox ClKind"
  Demux/3 -> BusCreator/3  "PTC_Cfg GearBox nFGears"
  Demux/4 -> BusCreator/4  "PTC_Cfg GearBox iFGear0"
  Demux/5 -> BusCreator/5  "PTC_Cfg GearBox iFGear1"
  Demux/6 -> BusCreator/6  "PTC_Cfg GearBox iFGear2"
  Demux/7 -> BusCreator/7  "PTC_Cfg GearBox iFGear3"
  Demux/8 -> BusCreator/8  "PTC_Cfg GearBox iFGear4"
  Demux/9 -> BusCreator/9  "PTC_Cfg GearBox iFGear5"
  Demux/10 -> BusCreator/10  "PTC_Cfg GearBox iFGear6"
  Demux/11 -> BusCreator/11  "PTC_Cfg GearBox iFGear7"
  Demux/12 -> BusCreator/12  "PTC_Cfg GearBox iFGear8"
  Demux/13 -> BusCreator/13  "PTC_Cfg GearBox iFGear9"
  Demux/14 -> BusCreator/14  "PTC_Cfg GearBox iFGear10"
  Demux/15 -> BusCreator/15  "PTC_Cfg GearBox iFGear11"
  Demux/16 -> BusCreator/16  "PTC_Cfg GearBox iFGear12"
  Demux/17 -> BusCreator/17  "PTC_Cfg GearBox iFGear13"
  Demux/18 -> BusCreator/18  "PTC_Cfg GearBox iFGear14"
  Demux/19 -> BusCreator/19  "PTC_Cfg GearBox iFGear15"
  Demux/20 -> BusCreator/20  "PTC_Cfg GearBox iFGear16"
  Demux/21 -> BusCreator/21  "PTC_Cfg GearBox nBGears"
  Demux/22 -> BusCreator/22  "PTC_Cfg GearBox iBGear0"
  Demux/23 -> BusCreator/23  "PTC_Cfg GearBox iBGear1"
  Demux/24 -> BusCreator/24  "PTC_Cfg GearBox iBGear2"
  Demux/25 -> BusCreator/25  "PTC_Cfg GearBox iBGear3"
  Demux/26 -> BusCreator/26  "PTC_Cfg GearBox iBGear4"
  Demux/27 -> BusCreator/27  "PTC_Cfg GearBox iBGear5"
  Demux/28 -> BusCreator/28  "PTC_Cfg GearBox iBGear6"
  Demux/29 -> BusCreator/29  "PTC_Cfg GearBox iBGear7"
  Demux/30 -> BusCreator/30  "PTC_Cfg GearBox iBGear8"
  Demux/31 -> BusCreator/31  "PTC_Cfg GearBox iBGear9"
  Demux/32 -> BusCreator/32  "PTC_Cfg GearBox iBGear10"
  Demux/33 -> BusCreator/33  "PTC_Cfg GearBox iBGear11"
  Demux/34 -> BusCreator/34  "PTC_Cfg GearBox iBGear12"
  Demux/35 -> BusCreator/35  "PTC_Cfg GearBox iBGear13"
  Demux/36 -> BusCreator/36  "PTC_Cfg GearBox iBGear14"
  Demux/37 -> BusCreator/37  "PTC_Cfg GearBox iBGear15"
  Demux/38 -> BusCreator/38  "PTC_Cfg GearBox iBGear16"

== system TorqueVect/CarMaker/IPG Vehicle/PowerTrain/PTControl Example/PTControl_In1/CreateBus PTC_Cfg GearBoxM0 ==
  In : Inport
  BusCreator : BusCreator  Inputs=38
  Demux : Demux  Outputs=38
      settings: DisplayOption=none
  Out : Outport  VectorParamsAs1DForOutWhenUnconnected=off
  wires:
  In/1 -> Demux/1
  BusCreator/1 -> Out/1
  Demux/1 -> BusCreator/1  "PTC_Cfg GearBoxM0 GBKind"
  Demux/2 -> BusCreator/2  "PTC_Cfg GearBoxM0 ClKind"
  Demux/3 -> BusCreator/3  "PTC_Cfg GearBoxM0 nFGears"
  Demux/4 -> BusCreator/4  "PTC_Cfg GearBoxM0 iFGear0"
  Demux/5 -> BusCreator/5  "PTC_Cfg GearBoxM0 iFGear1"
  Demux/6 -> BusCreator/6  "PTC_Cfg GearBoxM0 iFGear2"
  Demux/7 -> BusCreator/7  "PTC_Cfg GearBoxM0 iFGear3"
  Demux/8 -> BusCreator/8  "PTC_Cfg GearBoxM0 iFGear4"
  Demux/9 -> BusCreator/9  "PTC_Cfg GearBoxM0 iFGear5"
  Demux/10 -> BusCreator/10  "PTC_Cfg GearBoxM0 iFGear6"
  Demux/11 -> BusCreator/11  "PTC_Cfg GearBoxM0 iFGear7"
  Demux/12 -> BusCreator/12  "PTC_Cfg GearBoxM0 iFGear8"
  Demux/13 -> BusCreator/13  "PTC_Cfg GearBoxM0 iFGear9"
  Demux/14 -> BusCreator/14  "PTC_Cfg GearBoxM0 iFGear10"
  Demux/15 -> BusCreator/15  "PTC_Cfg GearBoxM0 iFGear11"
  Demux/16 -> BusCreator/16  "PTC_Cfg GearBoxM0 iFGear12"
  Demux/17 -> BusCreator/17  "PTC_Cfg GearBoxM0 iFGear13"
  Demux/18 -> BusCreator/18  "PTC_Cfg GearBoxM0 iFGear14"
  Demux/19 -> BusCreator/19  "PTC_Cfg GearBoxM0 iFGear15"
  Demux/20 -> BusCreator/20  "PTC_Cfg GearBoxM0 iFGear16"
  Demux/21 -> BusCreator/21  "PTC_Cfg GearBoxM0 nBGears"
  Demux/22 -> BusCreator/22  "PTC_Cfg GearBoxM0 iBGear0"
  Demux/23 -> BusCreator/23  "PTC_Cfg GearBoxM0 iBGear1"
  Demux/24 -> BusCreator/24  "PTC_Cfg GearBoxM0 iBGear2"
  Demux/25 -> BusCreator/25  "PTC_Cfg GearBoxM0 iBGear3"
  Demux/26 -> BusCreator/26  "PTC_Cfg GearBoxM0 iBGear4"
  Demux/27 -> BusCreator/27  "PTC_Cfg GearBoxM0 iBGear5"
  Demux/28 -> BusCreator/28  "PTC_Cfg GearBoxM0 iBGear6"
  Demux/29 -> BusCreator/29  "PTC_Cfg GearBoxM0 iBGear7"
  Demux/30 -> BusCreator/30  "PTC_Cfg GearBoxM0 iBGear8"
  Demux/31 -> BusCreator/31  "PTC_Cfg GearBoxM0 iBGear9"
  Demux/32 -> BusCreator/32  "PTC_Cfg GearBoxM0 iBGear10"
  Demux/33 -> BusCreator/33  "PTC_Cfg GearBoxM0 iBGear11"
  Demux/34 -> BusCreator/34  "PTC_Cfg GearBoxM0 iBGear12"
  Demux/35 -> BusCreator/35  "PTC_Cfg GearBoxM0 iBGear13"
  Demux/36 -> BusCreator/36  "PTC_Cfg GearBoxM0 iBGear14"
  Demux/37 -> BusCreator/37  "PTC_Cfg GearBoxM0 iBGear15"
  Demux/38 -> BusCreator/38  "PTC_Cfg GearBoxM0 iBGear16"

== system TorqueVect/CarMaker/IPG Vehicle/PowerTrain/PTControl Example/PTControl_In1/CreateBus PTC_Cfg GearBoxM1 ==
  In : Inport
  BusCreator : BusCreator  Inputs=38
  Demux : Demux  Outputs=38
      settings: DisplayOption=none
  Out : Outport  VectorParamsAs1DForOutWhenUnconnected=off
  wires:
  In/1 -> Demux/1
  BusCreator/1 -> Out/1
  Demux/1 -> BusCreator/1  "PTC_Cfg GearBoxM1 GBKind"
  Demux/2 -> BusCreator/2  "PTC_Cfg GearBoxM1 ClKind"
  Demux/3 -> BusCreator/3  "PTC_Cfg GearBoxM1 nFGears"
  Demux/4 -> BusCreator/4  "PTC_Cfg GearBoxM1 iFGear0"
  Demux/5 -> BusCreator/5  "PTC_Cfg GearBoxM1 iFGear1"
  Demux/6 -> BusCreator/6  "PTC_Cfg GearBoxM1 iFGear2"
  Demux/7 -> BusCreator/7  "PTC_Cfg GearBoxM1 iFGear3"
  Demux/8 -> BusCreator/8  "PTC_Cfg GearBoxM1 iFGear4"
  Demux/9 -> BusCreator/9  "PTC_Cfg GearBoxM1 iFGear5"
  Demux/10 -> BusCreator/10  "PTC_Cfg GearBoxM1 iFGear6"
  Demux/11 -> BusCreator/11  "PTC_Cfg GearBoxM1 iFGear7"
  Demux/12 -> BusCreator/12  "PTC_Cfg GearBoxM1 iFGear8"
  Demux/13 -> BusCreator/13  "PTC_Cfg GearBoxM1 iFGear9"
  Demux/14 -> BusCreator/14  "PTC_Cfg GearBoxM1 iFGear10"
  Demux/15 -> BusCreator/15  "PTC_Cfg GearBoxM1 iFGear11"
  Demux/16 -> BusCreator/16  "PTC_Cfg GearBoxM1 iFGear12"
  Demux/17 -> BusCreator/17  "PTC_Cfg GearBoxM1 iFGear13"
  Demux/18 -> BusCreator/18  "PTC_Cfg GearBoxM1 iFGear14"
  Demux/19 -> BusCreator/19  "PTC_Cfg GearBoxM1 iFGear15"
  Demux/20 -> BusCreator/20  "PTC_Cfg GearBoxM1 iFGear16"
  Demux/21 -> BusCreator/21  "PTC_Cfg GearBoxM1 nBGears"
  Demux/22 -> BusCreator/22  "PTC_Cfg GearBoxM1 iBGear0"
  Demux/23 -> BusCreator/23  "PTC_Cfg GearBoxM1 iBGear1"
  Demux/24 -> BusCreator/24  "PTC_Cfg GearBoxM1 iBGear2"
  Demux/25 -> BusCreator/25  "PTC_Cfg GearBoxM1 iBGear3"
  Demux/26 -> BusCreator/26  "PTC_Cfg GearBoxM1 iBGear4"
  Demux/27 -> BusCreator/27  "PTC_Cfg GearBoxM1 iBGear5"
  Demux/28 -> BusCreator/28  "PTC_Cfg GearBoxM1 iBGear6"
  Demux/29 -> BusCreator/29  "PTC_Cfg GearBoxM1 iBGear7"
  Demux/30 -> BusCreator/30  "PTC_Cfg GearBoxM1 iBGear8"
  Demux/31 -> BusCreator/31  "PTC_Cfg GearBoxM1 iBGear9"
  Demux/32 -> BusCreator/32  "PTC_Cfg GearBoxM1 iBGear10"
  Demux/33 -> BusCreator/33  "PTC_Cfg GearBoxM1 iBGear11"
  Demux/34 -> BusCreator/34  "PTC_Cfg GearBoxM1 iBGear12"
  Demux/35 -> BusCreator/35  "PTC_Cfg GearBoxM1 iBGear13"
  Demux/36 -> BusCreator/36  "PTC_Cfg GearBoxM1 iBGear14"
  Demux/37 -> BusCreator/37  "PTC_Cfg GearBoxM1 iBGear15"
  Demux/38 -> BusCreator/38  "PTC_Cfg GearBoxM1 iBGear16"

== system TorqueVect/CarMaker/IPG Vehicle/PowerTrain/PTControl Example/PTControl_In1/CreateBus PTC_Cfg GearBoxM2 ==
  In : Inport
  BusCreator : BusCreator  Inputs=38
  Demux : Demux  Outputs=38
      settings: DisplayOption=none
  Out : Outport  VectorParamsAs1DForOutWhenUnconnected=off
  wires:
  In/1 -> Demux/1
  BusCreator/1 -> Out/1
  Demux/1 -> BusCreator/1  "PTC_Cfg GearBoxM2 GBKind"
  Demux/2 -> BusCreator/2  "PTC_Cfg GearBoxM2 ClKind"
  Demux/3 -> BusCreator/3  "PTC_Cfg GearBoxM2 nFGears"
  Demux/4 -> BusCreator/4  "PTC_Cfg GearBoxM2 iFGear0"
  Demux/5 -> BusCreator/5  "PTC_Cfg GearBoxM2 iFGear1"
  Demux/6 -> BusCreator/6  "PTC_Cfg GearBoxM2 iFGear2"
  Demux/7 -> BusCreator/7  "PTC_Cfg GearBoxM2 iFGear3"
  Demux/8 -> BusCreator/8  "PTC_Cfg GearBoxM2 iFGear4"
  Demux/9 -> BusCreator/9  "PTC_Cfg GearBoxM2 iFGear5"
  Demux/10 -> BusCreator/10  "PTC_Cfg GearBoxM2 iFGear6"
  Demux/11 -> BusCreator/11  "PTC_Cfg GearBoxM2 iFGear7"
  Demux/12 -> BusCreator/12  "PTC_Cfg GearBoxM2 iFGear8"
  Demux/13 -> BusCreator/13  "PTC_Cfg GearBoxM2 iFGear9"
  Demux/14 -> BusCreator/14  "PTC_Cfg GearBoxM2 iFGear10"
  Demux/15 -> BusCreator/15  "PTC_Cfg GearBoxM2 iFGear11"
  Demux/16 -> BusCreator/16  "PTC_Cfg GearBoxM2 iFGear12"
  Demux/17 -> BusCreator/17  "PTC_Cfg GearBoxM2 iFGear13"
  Demux/18 -> BusCreator/18  "PTC_Cfg GearBoxM2 iFGear14"
  Demux/19 -> BusCreator/19  "PTC_Cfg GearBoxM2 iFGear15"
  Demux/20 -> BusCreator/20  "PTC_Cfg GearBoxM2 iFGear16"
  Demux/21 -> BusCreator/21  "PTC_Cfg GearBoxM2 nBGears"
  Demux/22 -> BusCreator/22  "PTC_Cfg GearBoxM2 iBGear0"
  Demux/23 -> BusCreator/23  "PTC_Cfg GearBoxM2 iBGear1"
  Demux/24 -> BusCreator/24  "PTC_Cfg GearBoxM2 iBGear2"
  Demux/25 -> BusCreator/25  "PTC_Cfg GearBoxM2 iBGear3"
  Demux/26 -> BusCreator/26  "PTC_Cfg GearBoxM2 iBGear4"
  Demux/27 -> BusCreator/27  "PTC_Cfg GearBoxM2 iBGear5"
  Demux/28 -> BusCreator/28  "PTC_Cfg GearBoxM2 iBGear6"
  Demux/29 -> BusCreator/29  "PTC_Cfg GearBoxM2 iBGear7"
  Demux/30 -> BusCreator/30  "PTC_Cfg GearBoxM2 iBGear8"
  Demux/31 -> BusCreator/31  "PTC_Cfg GearBoxM2 iBGear9"
  Demux/32 -> BusCreator/32  "PTC_Cfg GearBoxM2 iBGear10"
  Demux/33 -> BusCreator/33  "PTC_Cfg GearBoxM2 iBGear11"
  Demux/34 -> BusCreator/34  "PTC_Cfg GearBoxM2 iBGear12"
  Demux/35 -> BusCreator/35  "PTC_Cfg GearBoxM2 iBGear13"
  Demux/36 -> BusCreator/36  "PTC_Cfg GearBoxM2 iBGear14"
  Demux/37 -> BusCreator/37  "PTC_Cfg GearBoxM2 iBGear15"
  Demux/38 -> BusCreator/38  "PTC_Cfg GearBoxM2 iBGear16"

== system TorqueVect/CarMaker/IPG Vehicle/PowerTrain/PTControl Example/PTControl_In1/CreateBus PTC_Cfg GearBoxM3 ==
  In : Inport
  BusCreator : BusCreator  Inputs=38
  Demux : Demux  Outputs=38
      settings: DisplayOption=none
  Out : Outport  VectorParamsAs1DForOutWhenUnconnected=off
  wires:
  In/1 -> Demux/1
  BusCreator/1 -> Out/1
  Demux/1 -> BusCreator/1  "PTC_Cfg GearBoxM3 GBKind"
  Demux/2 -> BusCreator/2  "PTC_Cfg GearBoxM3 ClKind"
  Demux/3 -> BusCreator/3  "PTC_Cfg GearBoxM3 nFGears"
  Demux/4 -> BusCreator/4  "PTC_Cfg GearBoxM3 iFGear0"
  Demux/5 -> BusCreator/5  "PTC_Cfg GearBoxM3 iFGear1"
  Demux/6 -> BusCreator/6  "PTC_Cfg GearBoxM3 iFGear2"
  Demux/7 -> BusCreator/7  "PTC_Cfg GearBoxM3 iFGear3"
  Demux/8 -> BusCreator/8  "PTC_Cfg GearBoxM3 iFGear4"
  Demux/9 -> BusCreator/9  "PTC_Cfg GearBoxM3 iFGear5"
  Demux/10 -> BusCreator/10  "PTC_Cfg GearBoxM3 iFGear6"
  Demux/11 -> BusCreator/11  "PTC_Cfg GearBoxM3 iFGear7"
  Demux/12 -> BusCreator/12  "PTC_Cfg GearBoxM3 iFGear8"
  Demux/13 -> BusCreator/13  "PTC_Cfg GearBoxM3 iFGear9"
  Demux/14 -> BusCreator/14  "PTC_Cfg GearBoxM3 iFGear10"
  Demux/15 -> BusCreator/15  "PTC_Cfg GearBoxM3 iFGear11"
  Demux/16 -> BusCreator/16  "PTC_Cfg GearBoxM3 iFGear12"
  Demux/17 -> BusCreator/17  "PTC_Cfg GearBoxM3 iFGear13"
  Demux/18 -> BusCreator/18  "PTC_Cfg GearBoxM3 iFGear14"
  Demux/19 -> BusCreator/19  "PTC_Cfg GearBoxM3 iFGear15"
  Demux/20 -> BusCreator/20  "PTC_Cfg GearBoxM3 iFGear16"
  Demux/21 -> BusCreator/21  "PTC_Cfg GearBoxM3 nBGears"
  Demux/22 -> BusCreator/22  "PTC_Cfg GearBoxM3 iBGear0"
  Demux/23 -> BusCreator/23  "PTC_Cfg GearBoxM3 iBGear1"
  Demux/24 -> BusCreator/24  "PTC_Cfg GearBoxM3 iBGear2"
  Demux/25 -> BusCreator/25  "PTC_Cfg GearBoxM3 iBGear3"
  Demux/26 -> BusCreator/26  "PTC_Cfg GearBoxM3 iBGear4"
  Demux/27 -> BusCreator/27  "PTC_Cfg GearBoxM3 iBGear5"
  Demux/28 -> BusCreator/28  "PTC_Cfg GearBoxM3 iBGear6"
  Demux/29 -> BusCreator/29  "PTC_Cfg GearBoxM3 iBGear7"
  Demux/30 -> BusCreator/30  "PTC_Cfg GearBoxM3 iBGear8"
  Demux/31 -> BusCreator/31  "PTC_Cfg GearBoxM3 iBGear9"
  Demux/32 -> BusCreator/32  "PTC_Cfg GearBoxM3 iBGear10"
  Demux/33 -> BusCreator/33  "PTC_Cfg GearBoxM3 iBGear11"
  Demux/34 -> BusCreator/34  "PTC_Cfg GearBoxM3 iBGear12"
  Demux/35 -> BusCreator/35  "PTC_Cfg GearBoxM3 iBGear13"
  Demux/36 -> BusCreator/36  "PTC_Cfg GearBoxM3 iBGear14"
  Demux/37 -> BusCreator/37  "PTC_Cfg GearBoxM3 iBGear15"
  Demux/38 -> BusCreator/38  "PTC_Cfg GearBoxM3 iBGear16"

== system TorqueVect/CarMaker/IPG Vehicle/PowerTrain/PTControl Example/PTControl_In1/CreateBus PTC_Cfg ISG ==
  In : Inport
  BusCreator : BusCreator  Inputs=4
  Demux : Demux
      settings: DisplayOption=none
  Out : Outport  VectorParamsAs1DForOutWhenUnconnected=off
  wires:
  In/1 -> Demux/1
  BusCreator/1 -> Out/1
  Demux/1 -> BusCreator/1  "PTC_Cfg ISG Level"
  Demux/2 -> BusCreator/2  "PTC_Cfg ISG Ratio"
  Demux/3 -> BusCreator/3  "PTC_Cfg ISG rotv_Mot_max"
  Demux/4 -> BusCreator/4  "PTC_Cfg ISG rotv_Gen_max"

== system TorqueVect/CarMaker/IPG Vehicle/PowerTrain/PTControl Example/PTControl_In1/CreateBus PTC_Cfg Misc ==
  In : Inport
  BusCreator : BusCreator  Inputs=13
  Demux : Demux  Outputs=13
      settings: DisplayOption=none
  Out : Outport  VectorParamsAs1DForOutWhenUnconnected=off
  wires:
  In/1 -> Demux/1
  BusCreator/1 -> Out/1
  Demux/1 -> BusCreator/1  "PTC_Cfg PTKind"
  Demux/2 -> BusCreator/2  "PTC_Cfg ClKind"
  Demux/3 -> BusCreator/3  "PTC_Cfg nMotor"
  Demux/4 -> BusCreator/4  "PTC_Cfg nGearBoxM"
  Demux/5 -> BusCreator/5  "PTC_Cfg nPlanetGear"
  Demux/6 -> BusCreator/6  "PTC_Cfg Vehicle_nWheels"
  Demux/7 -> BusCreator/7  "PTC_Cfg WheelRadius"
  Demux/8 -> BusCreator/8  "PTC_Cfg Aero_Frcx"
  Demux/9 -> BusCreator/9  "PTC_Cfg DL_iDiff_mean"
  Demux/10 -> BusCreator/10  "PTC_Cfg DriveSourcePos0"
  Demux/11 -> BusCreator/11  "PTC_Cfg DriveSourcePos1"
  Demux/12 -> BusCreator/12  "PTC_Cfg DriveSourcePos2"
  Demux/13 -> BusCreator/13  "PTC_Cfg DriveSourcePos3"

== system TorqueVect/CarMaker/IPG Vehicle/PowerTrain/PTControl Example/PTControl_In1/CreateBus PTC_Cfg Motor ==
  In : Inport
  BusCreator : BusCreator  Inputs=16
  Demux : Demux  Outputs=16
      settings: DisplayOption=none
  Out : Outport  VectorParamsAs1DForOutWhenUnconnected=off
  wires:
  In/1 -> Demux/1
  BusCreator/1 -> Out/1
  Demux/1 -> BusCreator/1  "PTC_Cfg Motor0 Level"
  Demux/2 -> BusCreator/2  "PTC_Cfg Motor0 Ratio"
  Demux/3 -> BusCreator/3  "PTC_Cfg Motor0 rotv_Mot_max"
  Demux/4 -> BusCreator/4  "PTC_Cfg Motor0 rotv_Gen_max"
  Demux/5 -> BusCreator/5  "PTC_Cfg Motor1 Level"
  Demux/6 -> BusCreator/6  "PTC_Cfg Motor1 Ratio"
  Demux/7 -> BusCreator/7  "PTC_Cfg Motor1 rotv_Mot_max"
  Demux/8 -> BusCreator/8  "PTC_Cfg Motor1 rotv_Gen_max"
  Demux/9 -> BusCreator/9  "PTC_Cfg Motor2 Level"
  Demux/10 -> BusCreator/10  "PTC_Cfg Motor2 Ratio"
  Demux/11 -> BusCreator/11  "PTC_Cfg Motor2 rotv_Mot_max"
  Demux/12 -> BusCreator/12  "PTC_Cfg Motor2 rotv_Gen_max"
  Demux/13 -> BusCreator/13  "PTC_Cfg Motor3 Level"
  Demux/14 -> BusCreator/14  "PTC_Cfg Motor3 Ratio"
  Demux/15 -> BusCreator/15  "PTC_Cfg Motor3 rotv_Mot_max"
  Demux/16 -> BusCreator/16  "PTC_Cfg Motor3 rotv_Gen_max"

== system TorqueVect/CarMaker/IPG Vehicle/PowerTrain/PTControl Example/PTControl_In1/CreateBus PTC_Cfg PlanetGear ==
  In : Inport
  BusCreator : BusCreator  Inputs=1
  Demux : Demux  Outputs=1
      settings: DisplayOption=none
  Out : Outport  VectorParamsAs1DForOutWhenUnconnected=off
  wires:
  In/1 -> Demux/1
  BusCreator/1 -> Out/1
  Demux/1 -> BusCreator/1  "PTC_Cfg PlanetGear0 Ratio"
